simulink model "gm_MATLAB_TO_VHDL3_SIMULINK"  (R2018b)
settings: Solver=FixedStepAuto  StartTime=0.0  StopTime=10.0  FixedStep=0.01  RelTol=1e-3
undefined symbols (not defined in the file or in its folder): DiscIntNeverNeededParam
libraries: simulink x1
settings Model: Creator=ESPINO NOTEBOOK  LastModifiedBy=ESPINO NOTEBOOK
settings OptimizationCC: BlockReduction=off  ConditionallyExecuteInputs=off
settings DebuggingCC: InheritedTsInSrcMsg=none

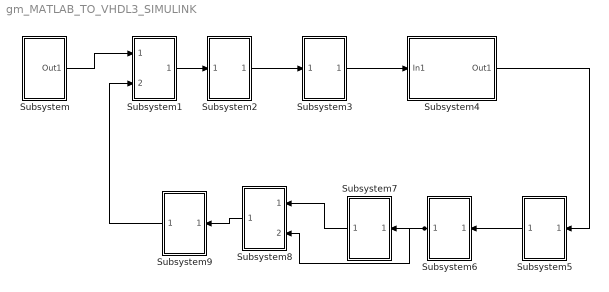
== system gm_MATLAB_TO_VHDL3_SIMULINK ==
  Subsystem : Subsystem
  Subsystem1 : Subsystem
  Subsystem2 : Subsystem
  Subsystem3 : Subsystem
  Subsystem4 : Subsystem
  Subsystem5 : Subsystem
  Subsystem6 : Subsystem
  Subsystem7 : Subsystem
  Subsystem8 : Subsystem
  Subsystem9 : Subsystem
  wires:
  Subsystem/1(Out1) -> Subsystem1/1(In1)
  Subsystem9/1(Out1) -> Subsystem1/2(In2)
  Subsystem8/1(Out1) -> Subsystem9/1(In1)
  Subsystem7/1(Out1) -> Subsystem8/1(In1)
  Subsystem5/1(Out1) -> Subsystem6/1(In1)
  Subsystem6/1(Out1) -> Subsystem7/1(In1), Subsystem8/2(In2)
  Subsystem4/1(Out1) -> Subsystem5/1(In1)
  Subsystem3/1(Out1) -> Subsystem4/1(In1)
  Subsystem2/1(Out1) -> Subsystem3/1(In1)
  Subsystem1/1(Out1) -> Subsystem2/1(In1)

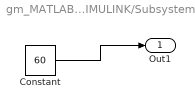
== system gm_MATLAB_TO_VHDL3_SIMULINK/Subsystem ==
  Constant : Constant  Value=60  SampleTime=0.01
  Out1 : Outport
  wires:
  Constant/1 -> Out1/1

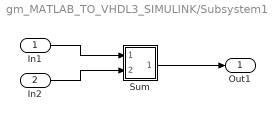
== system gm_MATLAB_TO_VHDL3_SIMULINK/Subsystem1 ==
  In1 : Inport  OutDataTypeStr=double  PortDimensions=1  SampleTime=0.01
  In2 : Inport  Port=2  OutDataTypeStr=double  PortDimensions=1  SampleTime=0.01
  Sum : Subsystem
      mask Display: disp('NFP\nadd');
  Out1 : Outport
  wires:
  In1/1 -> Sum/1(In1)
  In2/1 -> Sum/2(In2)
  Sum/1(Out1) -> Out1/1

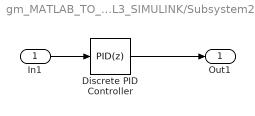
== system gm_MATLAB_TO_VHDL3_SIMULINK/Subsystem2 ==
  In1 : Inport
  Discrete PID Controller : simulink/Continuous/PID Controller  Controller=PID  Form=Parallel  TimeDomain=Discrete-time  SampleTime=0.01  IntegratorMethod=Forward Euler  FilterMethod=Forward Euler  ControllerParametersSource=internal  P=0.0223573377854503  I=0.126914026258104  D=0.000583636498025721  UseFilter=on  N=24.7802164814205  TunerSelectOption=Transfer Function Based (PID Tuner App)  InitialConditionSource=internal  InitialConditionForIntegrator=0  InitialConditionForFilter=0  DifferentiatorICPrevScaledInput=0  ExternalReset=none  TrackingMode=off  Kt=1  LimitOutput=off  UpperSaturationLimit=inf  LowerSaturationLimit=-inf  LinearizeAsGain=off  AntiWindupMode=none  Kb=1  POutMin=[]  POutMax=[]  IOutMin=[]  IOutMax=[]  DOutMin=[]  DOutMax=[]  NOutMin=[]  NOutMax=[]  SumOutMin=[]  SumOutMax=[]  SaturationOutMin=[]  SaturationOutMax=[]  PParamMin=[]  PParamMax=[]  IParamMin=[]  IParamMax=[]  DParamMin=[]  DParamMax=[]  NParamMin=[]  NParamMax=[]  KbParamMin=[]  KbParamMax=[]  KtParamMin=[]  KtParamMax=[]  KbOutMin=[]  KbOutMax=[]  KtOutMin=[]  KtOutMax=[]  IntegratorOutMin=[]  IntegratorOutMax=[]  FilterOutMin=[]  FilterOutMax=[]  SumI1OutMin=[]  SumI1OutMax=[]  SumI2OutMin=[]  SumI2OutMax=[]  SumI3OutMin=[]  SumI3OutMax=[]  SumI4OutMin=[]  SumI4OutMax=[]  SumDOutMin=[]  SumDOutMax=[]  DifferentiatorOutMin=[]  DifferentiatorOutMax=[]  FilterDiffOutCoefMin=[]  FilterDiffOutCoefMax=[]  ReciprocalOutMin=[]  ReciprocalOutMax=[]  SumDenOutMin=[]  SumDenOutMax=[]  SumNumOutMin=[]  SumNumOutMax=[]  DivideOutMin=[]  DivideOutMax=[]  IntegratorContinuousStateAttributes=''  IntegratorStateMustResolveToSignalObject=off  IntegratorRTWStateStorageClass=Auto  FilterContinuousStateAttributes=''  FilterStateMustResolveToSignalObject=off  FilterRTWStateStorageClass=Auto  ParallelPVariant=InternalParameters  IdealPVariant=Disabled  IVariant=InternalParameters  DVariant=InternalParameters  IntegratorVariant=Discrete  SatVariant=Disabled  AWVariant=Passthrough  PCopyVariant=Disabled  TRVariant=Disabled  FdbkBlocksVariant=Forward  IdealPFdbkVariant=Disabled  SatFdbkVariant=Disabled  DerivativeFilterVariant=ForwardEulerFilter  NVariant=InternalParameters  NCopyVariant=Disabled  FilterICVariant=InternalICsFilter  IntegratorICVariant=InternalICs  ExternalResetVariant=Disabled  TRSumVariant=Passthrough  SumFdbkVariant=Disabled  SumVariant=Sum_PID
  Out1 : Outport
  wires:
  In1/1 -> Discrete PID Controller/1
  Discrete PID Controller/1 -> Out1/1

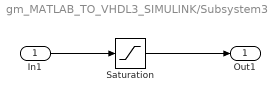
== system gm_MATLAB_TO_VHDL3_SIMULINK/Subsystem3 ==
  In1 : Inport
  Saturation : Saturate  UpperLimit=100  LowerLimit=0
  Out1 : Outport
  wires:
  In1/1 -> Saturation/1
  Saturation/1 -> Out1/1

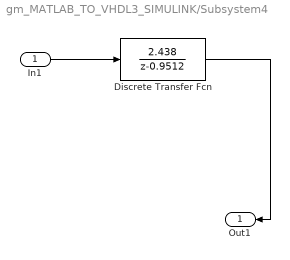
== system gm_MATLAB_TO_VHDL3_SIMULINK/Subsystem4 ==
  In1 : Inport
  Discrete Transfer Fcn : DiscreteTransferFcn  Numerator=[2.438]  Denominator=[1 -0.9512]  SampleTime=0.01
  Out1 : Outport
  wires:
  Discrete Transfer Fcn/1 -> Out1/1
  In1/1 -> Discrete Transfer Fcn/1

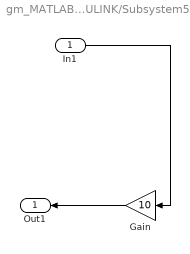
== system gm_MATLAB_TO_VHDL3_SIMULINK/Subsystem5 ==
  In1 : Inport
  Gain : Gain  Gain=10
  Out1 : Outport
  wires:
  In1/1 -> Gain/1
  Gain/1 -> Out1/1

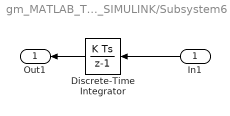
== system gm_MATLAB_TO_VHDL3_SIMULINK/Subsystem6 ==
  In1 : Inport
  Discrete-Time Integrator : DiscreteIntegrator  SampleTime=0.01  ICPrevOutput=DiscIntNeverNeededParam  ICPrevScaledInput=DiscIntNeverNeededParam
  Out1 : Outport
  wires:
  In1/1 -> Discrete-Time Integrator/1
  Discrete-Time Integrator/1 -> Out1/1

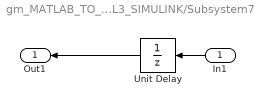
== system gm_MATLAB_TO_VHDL3_SIMULINK/Subsystem7 ==
  In1 : Inport
  Unit Delay : UnitDelay  SampleTime=0.01
  Out1 : Outport
  wires:
  Unit Delay/1 -> Out1/1
  In1/1 -> Unit Delay/1

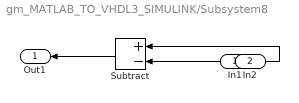
== system gm_MATLAB_TO_VHDL3_SIMULINK/Subsystem8 ==
  In1 : Inport
  In2 : Inport  Port=2
  Subtract : Sum  Inputs=+-
  Out1 : Outport
  wires:
  In1/1 -> Subtract/2
  Subtract/1 -> Out1/1
  In2/1 -> Subtract/1

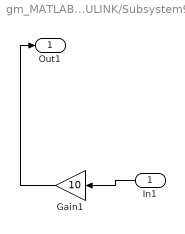
== system gm_MATLAB_TO_VHDL3_SIMULINK/Subsystem9 ==
  In1 : Inport
  Gain1 : Gain  Gain=10
  Out1 : Outport
  wires:
  Gain1/1 -> Out1/1
  In1/1 -> Gain1/1

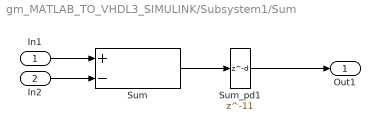
== system gm_MATLAB_TO_VHDL3_SIMULINK/Subsystem1/Sum ==
  In1 : Inport
  In2 : Inport  Port=2
  Sum : Sum  Inputs=+-  OutDataTypeStr=double  SampleTime=0.01  SaturateOnIntegerOverflow=on  InputSameDT=on
  Sum_pd1 : Delay  DelayLength=11  InputProcessing=Inherited
  Out1 : Outport
  wires:
  In1/1 -> Sum/1
  In2/1 -> Sum/2
  Sum/1 -> Sum_pd1/1
  Sum_pd1/1 -> Out1/1
